simulink model "z54_tran_2"  (R2015a)
settings: Solver=FixedStepDiscrete  StartTime=0.0  StopTime=99.0  FixedStep=1  RelTol=1e-3
settings Model: Creator=Bojana Vasic  LastModifiedBy=Bojana Vasic

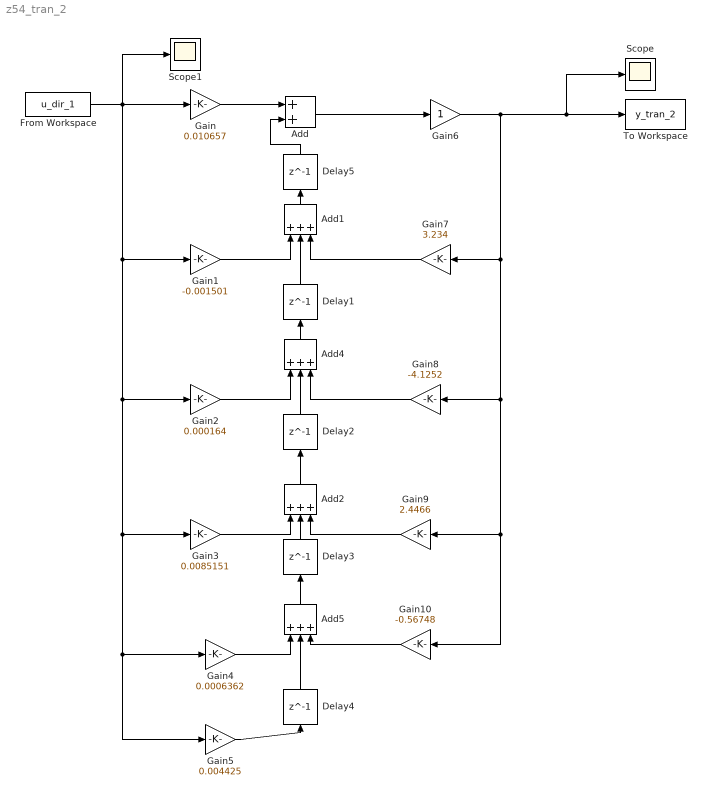
== system z54_tran_2 ==
  Add : Sum
  Add{1..2,4..5} (4 alike) : Sum  Inputs=+++
  Delay{1..5} (5 alike) : Delay  DelayLength=1
  From Workspace : FromWorkspace  VariableName=u_dir_1  SampleTime=1
  Gain : Gain  Gain=0.010657
  Gain1 : Gain  Gain=-0.001501
  Gain10 : Gain  Gain=-0.56748
  Gain2 : Gain  Gain=0.000164
  Gain3 : Gain  Gain=0.0085151
  Gain4 : Gain  Gain=0.0006362
  Gain5 : Gain  Gain=0.004425
  Gain6 : Gain
  Gain7 : Gain  Gain=3.234
  Gain8 : Gain  Gain=-4.1252
  Gain9 : Gain  Gain=2.4466
  Scope : Scope
  Scope1 : Scope
  To Workspace : ToWorkspace  VariableName=y_tran_2  SampleTime=-1
      settings: Save2DSignal=2-D array (concatenate along first dimension)
  wires:
  From Workspace/1 -> Gain5/1, Gain4/1, Gain3/1, Gain2/1, Gain1/1, Gain/1, Scope1/1
  Gain1/1 -> Add1/1
  Gain/1 -> Add/1
  Gain3/1 -> Add2/1
  Gain2/1 -> Add4/1
  Gain6/1 -> Gain10/1, Gain9/1, Gain8/1, Gain7/1, To Workspace/1, Scope/1
  Gain4/1 -> Add5/1
  Add1/1 -> Delay5/1
  Delay1/1 -> Add1/2
  Add4/1 -> Delay1/1
  Delay3/1 -> Add2/2
  Add2/1 -> Delay2/1
  Delay4/1 -> Add5/2
  Gain5/1 -> Delay4/1
  Delay2/1 -> Add4/2
  Delay5/1 -> Add/2
  Gain7/1 -> Add1/3
  Gain8/1 -> Add4/3
  Add/1 -> Gain6/1
  Gain9/1 -> Add2/3
  Gain10/1 -> Add5/3
  Add5/1 -> Delay3/1
